simulink model "Pendulo3D"  (R2015a)
settings: Solver=ode45  StartTime=0.0  StopTime=10.0  RelTol=1e-3
undefined symbols (not defined in the file): B, g, J, l, m
libraries: vrlib x1
settings Model: Creator=Henry Alberto  LastModifiedBy=Henry Alberto

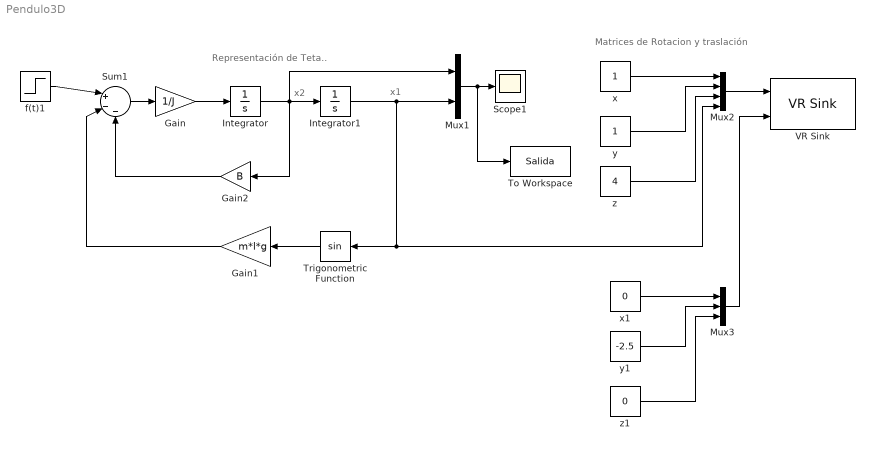
== system Pendulo3D ==
  note: Matrices de Rotacion y traslación
  note: x1
  note: x2
  note: Representación de Teta..
  Gain : Gain  Gain=1/J
  Gain1 : Gain  Gain=m*l*g
  Gain2 : Gain  Gain=B
  Integrator : Integrator
  Integrator1 : Integrator
  Mux1 : Mux  Inputs=2
  Mux2 : Mux
  Mux3 : Mux  Inputs=3
  Scope1 : Scope
  Sum1 : Sum  Inputs=|+--
  To Workspace : ToWorkspace  VariableName=Salida  SaveFormat=Timeseries  SampleTime=-1
  Trigonometric Function : Trigonometry
  VR Sink : vrlib/VR Sink  InstantiateOnLoad=on  SampleTime=0.1  ViewEnable=on  RemoteChange=off  RemoteView=off  FieldsWritten=Cable.rotation.4.1.1.double#Cable.translation.3.1.1.double  WorldFileName=Pendulo.WRL  AutoView=off  VideoDimensions=[]  AllowVariableSize=off
  f(t)1 : Step  Time=2  SampleTime=0
  x : Constant
  x1 : Constant  Value=0
  y : Constant
  y1 : Constant  Value=-2.5
  z : Constant  Value=4
  z1 : Constant  Value=0
  wires:
  Sum1/1 -> Gain/1
  Gain/1 -> Integrator/1
  Integrator/1 -> Mux1/1, Gain2/1, Integrator1/1
  Trigonometric Function/1 -> Gain1/1
  Gain2/1 -> Sum1/3
  Gain1/1 -> Sum1/2
  f(t)1/1 -> Sum1/1
  Mux1/1 -> To Workspace/1, Scope1/1
  x/1 -> Mux2/1
  y/1 -> Mux2/2
  z/1 -> Mux2/3
  x1/1 -> Mux3/1
  y1/1 -> Mux3/2
  z1/1 -> Mux3/3
  Mux3/1 -> VR Sink/2
  Mux2/1 -> VR Sink/1
  Integrator1/1 -> Mux2/4, Trigonometric Function/1, Mux1/2
